simulink library "library"  (Simulink 7.6)
settings: Solver=ode45  StartTime=0.0  StopTime=10.0  RelTol=1e-3
undefined symbols (not defined in the file or in its folder): data_rate, fc
libraries: simulink x2, dspsrcs4 x2, commrandsrc2 x1
settings Model: Creator=XARA  LastModifiedBy=XARA

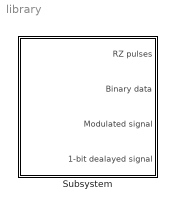
== system library ==
  Subsystem : Subsystem  mask(OOK modulated RZ pulses){data_rate=4, Am1=1, Am2=1, fc=50*data_rate, f=2, sample_time=1/(2*100*fc)}
      mask prompts: data_rate "Data rate in bits/s"; Am1 "Amplitude 1"; Am2 "Amplitude 2"; fc "Carrier frequency in Hz"; f "Frequency of second"
      mask help: This subsystem outputs RZ pulses as well as OOK modulated pulses

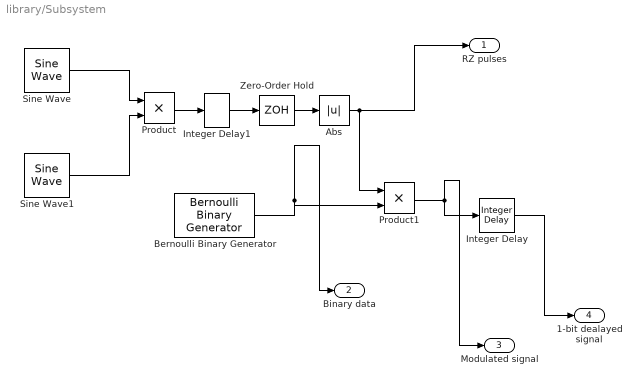
== system library/Subsystem ==
  Abs : Abs
  Bernoulli Binary Generator : commrandsrc2/Bernoulli Binary Generator  DialogController=commDDGCreate  DialogControllerArgs=DataTag0  SystemSampleTime=-1  P=0.5  seed=61  Ts=1/data_rate  frameBased=off  sampPerFrame=1  orient=off  outDataType=double
  Integer Delay : simulink/Discrete/Integer Delay  NumDelays=50  vinit=0.0  samptime=-1
  Integer Delay1 : simulink/Discrete/Integer Delay  NumDelays=5000  vinit=0.0  samptime=-1
  Product : Product  RndMeth=Zero
  Product1 : Product  RndMeth=Zero
  Sine Wave : dspsrcs4/Sine Wave  Amplitude=Am1  Frequency=fc  Phase=pi/2  SampleMode=Discrete  OutComplex=Real  CompMethod=Trigonometric fcn  TableSize=Speed  SampleTime=sample_time  SamplesPerFrame=1  ResetState=Restart at time zero  dataType=double  wordLen=16  udDataType=sfix(16)  fracBitsMode=Best precision  numFracBits=15  OutDataTypeStr=double  LastOutDataTypeStr=double
  Sine Wave1 : dspsrcs4/Sine Wave  Amplitude=Am2  Frequency=f  Phase=pi/2  SampleMode=Discrete  OutComplex=Real  CompMethod=Trigonometric fcn  TableSize=Speed  SampleTime=sample_time  SamplesPerFrame=1  ResetState=Restart at time zero  dataType=double  wordLen=16  udDataType=sfix(16)  fracBitsMode=Best precision  numFracBits=15  OutDataTypeStr=double  LastOutDataTypeStr=double
  Zero-Order Hold : ZeroOrderHold  SampleTime=1/200
  RZ pulses : Outport
  Binary data : Outport  Port=2
  Modulated signal : Outport  Port=3
  1-bit dealayed signal : Outport  Port=4
  wires:
  Integer Delay1/1 -> Zero-Order Hold/1
  Integer Delay/1 -> 1-bit dealayed signal/1
  Product1/1 -> Integer Delay/1, Modulated signal/1
  Bernoulli Binary Generator/1 -> Product1/2, Binary data/1
  Abs/1 -> Product1/1, RZ pulses/1
  Zero-Order Hold/1 -> Abs/1
  Sine Wave1/1 -> Product/2
  Sine Wave/1 -> Product/1
  Product/1 -> Integer Delay1/1
